simulink model "gibalo_nonlinear_LQR"  (R2018a)
settings: Solver=ode45  StartTime=0.0  StopTime=10  RelTol=1e-3  EnableMultiTasking=on
values from neighbouring files (symbols this model uses):
  g = 9.81    [gibalo_system_model.m]
  J_bz = 8922223.33e-9 + m_b*l^2    (= 0.0139543664174)    [gibalo_system_model.m]
  Kr = -lqrd(G.a,G.b,Qd,Rd,Ts)    [gibalo_system_model.m]
  l = 0.06721    [gibalo_system_model.m]
  m_b = 1.114    [gibalo_system_model.m]
  MAX_ACCEL = inf    [gibalo_system_model.m]
  Ts = 0.005    [gibalo_system_model.m]
settings Model: Creator=antun  LastModifiedBy=Gospar
settings DataIOCC: LimitDataPoints=on  SaveFormat=Array
settings OptimizationCC: LifeSpan=inf
settings DebuggingCC: SFUnexpectedBacktrackingDiag=warning  SFNoUnconditionalDefaultTransitionDiag=warning  SFExecutionAtInitializationDiag=none
settings HardwareCC: ProdBitPerPointer=32  ProdBitPerSizeT=32  ProdBitPerPtrDiffT=32  ProdLargestAtomicFloat=None  ProdIntDivRoundTo=Undefined  ProdEndianess=Unspecified  ProdWordSize=32  ProdHWDeviceType=32-bit Generic
settings ModelReferenceCC: PropagateSignalLabelsOutOfModel=off
settings CodeAppCC: StateflowObjectComments=on
settings GRTTargetCC: TargetLangStandard=C89/C90 (ANSI)  GeneratePreprocessorConditionals=Disable all
settings ConfigComp: CovMetricSettings=dw  CovHtmlReporting=on  CovSaveCumulativeToWorkspaceVar=on  CovSaveSingleToWorkspaceVar=on  CovExternalEMLEnable=off

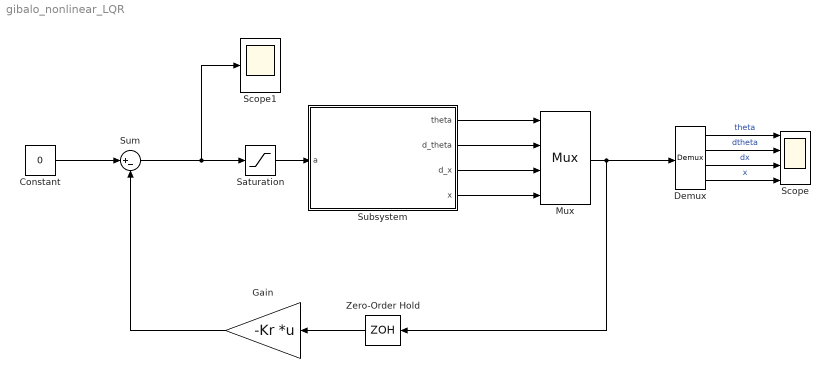
== system gibalo_nonlinear_LQR ==
  Constant : Constant  Value=0
  Demux : Demux
  Gain : Gain  Gain=-Kr  Multiplication=Matrix(K*u) (u vector)
  Mux : Mux
      settings: DisplayOption=signals
  Saturation : Saturate  UpperLimit=MAX_ACCEL  LowerLimit=-MAX_ACCEL
  Scope : Scope  NumInputPorts=4
  Scope1 : Scope
  Subsystem : Subsystem
  Sum : Sum  Inputs=|+-
  Zero-Order Hold : ZeroOrderHold  SampleTime=Ts
  wires:
  Saturation/1 -> Subsystem/1(a)
  Subsystem/1(theta) -> Mux/1
  Subsystem/2(d_theta) -> Mux/2
  Sum/1 -> Scope1/1, Saturation/1
  Gain/1 -> Sum/2
  Constant/1 -> Sum/1
  Mux/1 -> Zero-Order Hold/1, Demux/1
  Demux/1 -> Scope/1  "theta"
  Demux/2 -> Scope/2  "dtheta"
  Demux/3 -> Scope/3  "dx"
  Demux/4 -> Scope/4  "x"
  Subsystem/3(d_x) -> Mux/3
  Subsystem/4(x) -> Mux/4
  Zero-Order Hold/1 -> Gain/1

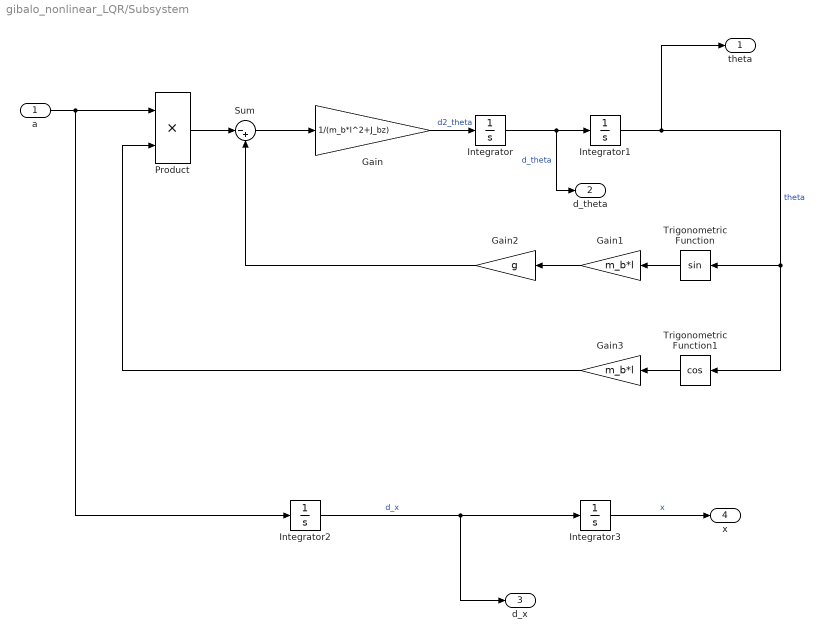
== system gibalo_nonlinear_LQR/Subsystem ==
  a : Inport
  Gain : Gain  Gain=1/(m_b*l^2+J_bz)
  Gain1 : Gain  Gain=m_b*l
  Gain2 : Gain  Gain=g
  Gain3 : Gain  Gain=m_b*l
  Integrator : Integrator
  Integrator1 : Integrator  InitialCondition=pi/30
  Integrator2 : Integrator
  Integrator3 : Integrator
  Product : Product
  Sum : Sum  Inputs=|-+
  Trigonometric Function : Trigonometry
  Trigonometric Function1 : Trigonometry  Operator=cos
  theta : Outport  PortDimensions=1
  d_theta : Outport  Port=2  PortDimensions=1
  d_x : Outport  Port=3
  x : Outport  Port=4
  wires:
  Gain/1 -> Integrator/1  "d2_theta"
  Product/1 -> Sum/1
  Gain2/1 -> Sum/2
  Integrator1/1 -> Trigonometric Function/1, Trigonometric Function1/1, theta/1  "theta"
  Trigonometric Function1/1 -> Gain3/1
  Integrator/1 -> d_theta/1, Integrator1/1  "d_theta"
  Sum/1 -> Gain/1
  Trigonometric Function/1 -> Gain1/1
  Integrator2/1 -> d_x/1, Integrator3/1  "d_x"
  a/1 -> Integrator2/1, Product/1
  Integrator3/1 -> x/1  "x"
  Gain1/1 -> Gain2/1
  Gain3/1 -> Product/2
